simulink subsystem "ctrl_ez_sub"  (R2024b)
settings: Solver=VariableStepAuto  StartTime=0.0  StopTime=10.0  RelTol=1e-3
values from neighbouring files (symbols this model uses):
  t_ss = tsw/30    (= 5.12820512821e-07)    [fidelity_pfc_vals.m]
  tsw = 1/(fsw*1e3)    (= 1.53846153846e-05)    [fidelity_pfc_vals.m]
undefined symbols (not defined in the file or in its folder): Discrete, Fc, spsSVPWMGenerator2LevelModel
libraries: mcbcontrolslib x5, slpidlib x4, simulink x4, simulink_extras x1, dspswit3 x1
settings Model: Creator=Angel  LastModifiedBy=Angel

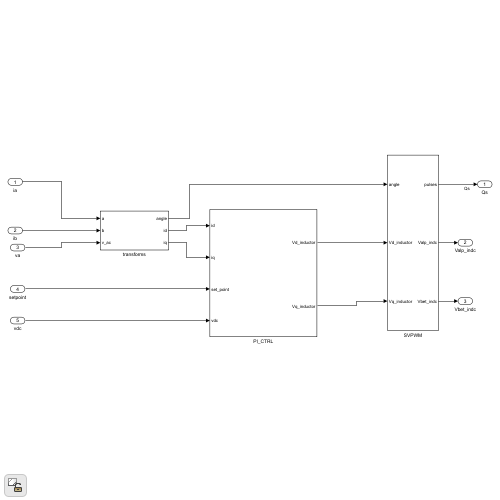
[thumbnail: Simulink's stored preview of the top-level diagram]
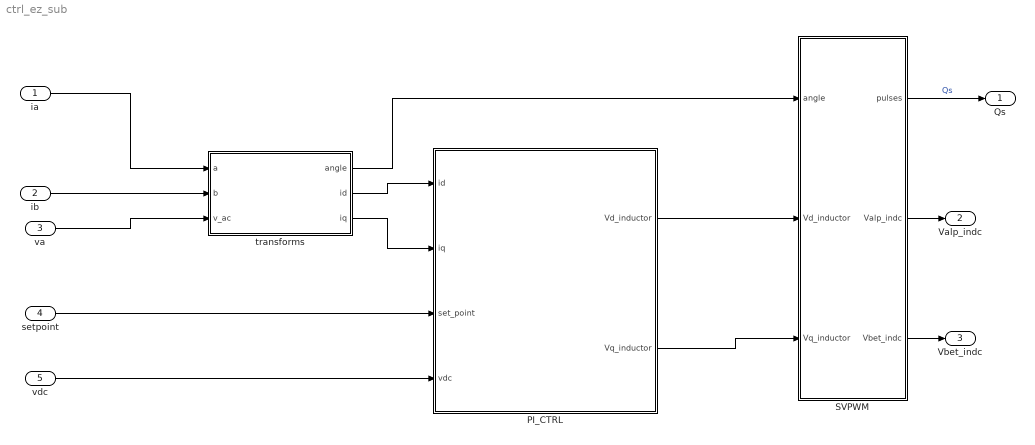
== system ctrl_ez_sub ==
  ia : Inport  OutDataTypeStr=single
  ib : Inport  Port=2  OutDataTypeStr=single
  va : Inport  Port=3  OutDataTypeStr=single
  setpoint : Inport  Port=4  OutDataTypeStr=single
  vdc : Inport  Port=5  OutDataTypeStr=single
  PI_CTRL : Subsystem  SystemSampleTime=tsw
  SVPWM : Subsystem  SystemSampleTime=tsw
  transforms : Subsystem  SystemSampleTime=tsw
  Qs : Outport
  Valp_indc : Outport  Port=2
  Vbet_indc : Outport  Port=3
  wires:
  SVPWM/1(pulses) -> Qs/1  "Qs"
  PI_CTRL/2(Vq_inductor) -> SVPWM/3(Vq_inductor)
  PI_CTRL/1(Vd_inductor) -> SVPWM/2(Vd_inductor)
  setpoint/1 -> PI_CTRL/3(set_point)
  transforms/2(id) -> PI_CTRL/1(id)
  transforms/1(angle) -> SVPWM/1(angle)
  transforms/3(iq) -> PI_CTRL/2(iq)
  va/1 -> transforms/3(v_ac)
  ib/1 -> transforms/2(b)
  ia/1 -> transforms/1(a)
  vdc/1 -> PI_CTRL/4(vdc)
  SVPWM/3(Vbet_indc) -> Vbet_indc/1
  SVPWM/2(Valp_indc) -> Valp_indc/1

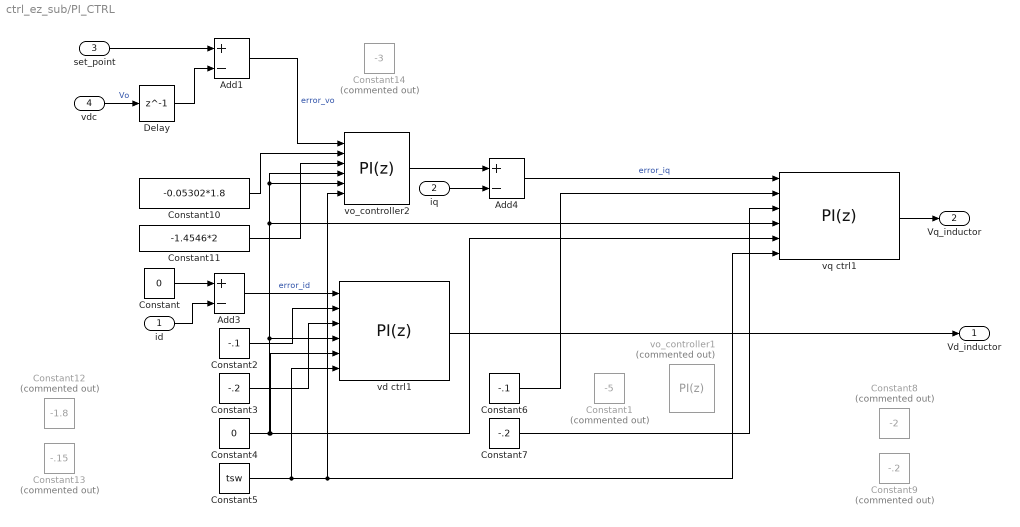
== system ctrl_ez_sub/PI_CTRL ==
  id : Inport
  iq : Inport  Port=2  OutDataTypeStr=single
  set_point : Inport  Port=3
  vdc : Inport  Port=4
  Add1 : Sum  Inputs=+-
  Add3 : Sum  Inputs=+-
  Add4 : Sum  Inputs=+-
  Constant : Constant  Value=0  OutDataTypeStr=single  SampleTime=-1
  Constant1 : Constant  Commented=on  Value=-5  SampleTime=t_ss
  Constant10 : Constant  Value=-0.05302*1.8  OutDataTypeStr=single  SampleTime=-1
  Constant11 : Constant  Value=-1.4546*2  OutDataTypeStr=single  SampleTime=-1
  Constant12 : Constant  Commented=on  Value=-1.8  OutDataTypeStr=single  SampleTime=-1
  Constant13 : Constant  Commented=on  Value=-.15  OutDataTypeStr=single  SampleTime=-1
  Constant14 : Constant  Commented=on  Value=-3  OutDataTypeStr=single  SampleTime=-1
  Constant2 : Constant  Value=-.1  OutDataTypeStr=single  SampleTime=-1
  Constant3 : Constant  Value=-.2  OutDataTypeStr=single  SampleTime=-1
  Constant4 : Constant  Value=0  OutDataTypeStr=single  SampleTime=-1
  Constant5 : Constant  Value=tsw  OutDataTypeStr=single  SampleTime=-1
  Constant6 : Constant  Value=-.1  OutDataTypeStr=single  SampleTime=-1
  Constant7 : Constant  Value=-.2  OutDataTypeStr=single  SampleTime=-1
  Constant8 : Constant  Commented=on  Value=-2  OutDataTypeStr=single  SampleTime=-1
  Constant9 : Constant  Commented=on  Value=-.2  OutDataTypeStr=single  SampleTime=-1
  Delay : Delay  DelayLength=1  InitialCondition=580
  "vd ctrl1 " : slpidlib/PID Controller  Controller=PI  Form=Parallel  TimeDomain=Discrete-time  UseExternalTs=on  SampleTime=-1  IntegratorMethod=Forward Euler  FilterMethod=Forward Euler  ControllerParametersSource=external  P=1  I=1  UseKiTs=off  D=0  UseExternalDerivativeSource=off  N=100  UseFilter=on  TunerSelectOption=Transfer Function Based (PID Tuner App)  ZeroCross=off  InitialConditionSource=external  InitialConditionForIntegrator=0  InitialConditionForFilter=0  DifferentiatorICPrevScaledInput=0  ExternalReset=level  TrackingMode=off  Kt=1  LimitOutput=on  SatLimitsSource=internal  UpperSaturationLimit=50  LowerSaturationLimit=-50  LinearizeAsGain=on  AntiWindupMode=clamping  Kb=1  LimitIntegrator=off  UpperIntegratorSaturationLimit=inf  LowerIntegratorSaturationLimit=-inf  RndMeth=Simplest  POutMin=[]  POutMax=[]  IOutMin=[]  IOutMax=[]  DOutMin=[]  DOutMax=[]  NOutMin=[]  NOutMax=[]  SumOutMin=[]  SumOutMax=[]  SaturationOutDataTypeStr=Inherit: Inherit via back propagation  SaturationOutMin=[]  SaturationOutMax=[]  PParamMin=[]  PParamMax=[]  IParamMin=[]  IParamMax=[]  DParamMin=[]  DParamMax=[]  NParamMin=[]  NParamMax=[]  KbParamMin=[]  KbParamMax=[]  KtParamMin=[]  KtParamMax=[]  KbOutMin=[]  KbOutMax=[]  KtOutMin=[]  KtOutMax=[]  IntegratorOutMin=[]  IntegratorOutMax=[]  FilterOutMin=[]  FilterOutMax=[]  SumI1OutMin=[]  SumI1OutMax=[]  SumI2OutMin=[]  SumI2OutMax=[]  SumI3OutMin=[]  SumI3OutMax=[]  SumI4OutMin=[]  SumI4OutMax=[]  SumDOutMin=[]  SumDOutMax=[]  DifferentiatorOutMin=[]  DifferentiatorOutMax=[]  FilterDiffOutCoefMin=[]  FilterDiffOutCoefMax=[]  ReciprocalOutMin=[]  ReciprocalOutMax=[]  SumDenOutMin=[]  SumDenOutMax=[]  SumNumOutMin=[]  SumNumOutMax=[]  DivideOutMin=[]  DivideOutMax=[]  UdiffTsProdOutMin=[]  UdiffTsProdOutMax=[]  NTsProdOutMin=[]  NTsProdOutMax=[]  UintegralTsProdOutMin=[]  UintegralTsProdOutMax=[]  UngainTsProdOutMin=[]  UngainTsProdOutMax=[]  ClampingZeroOutDataTypeStr=Inherit: Inherit via back propagation  ClampingZeroOutMin=[]  ClampingZeroOutMax=[]  FilterDenConstantOutDataTypeStr=Inherit: Inherit via back propagation  FilterDenConstantOutMin=[]  FilterDenConstantOutMax=[]  PCopyOutDataTypeStr=Inherit: Inherit via back propagation  PCopyOutMin=[]  PCopyOutMax=[]  NCopyOutDataTypeStr=Inherit: Inherit via back propagation  NCopyOutMin=[]  NCopyOutMax=[]  IntegratorContinuousStateAttributes=''  IntegratorStateMustResolveToSignalObject=off  IntegratorRTWStateStorageClass=Auto  FilterContinuousStateAttributes=''  FilterStateMustResolveToSignalObject=off  FilterRTWStateStorageClass=Auto  ParallelPVariant=ExternalParameters  IdealPVariant=Disabled  IVariant=ExternalParameters  DVariant=Disabled  IntegratorVariant=Discrete  SatVariant=Enabled  AWVariant=DiscClampingParallel  PCopyVariant=Disabled  TRVariant=Disabled  FdbkBlocksVariant=Forward  IdealPFdbkVariant=Disabled  SatFdbkVariant=Disabled  DerivativeFilterVariant=Disabled  NVariant=Disabled  NCopyVariant=Disabled_SignalSpec  FilterICVariant=Disabled  IntegratorICVariant=ExternalICs  ExternalResetVariant=ExternalReset  TRSumVariant=Passthrough  SumFdbkVariant=Disabled  SumVariant=Sum_PI  TsampFilterVariant=InternalTs  TsampNgainVariant=Passthrough  TsampIntegralVariant=ExternalTs  ExternalSaturationOutDataTypeStr=Inherit: Same as second input  DerivativeSourceVariant=Disabled  PreIntVariant=InternalPreInt
  vo_controller1 : slpidlib/PID Controller  Commented=on  Controller=PI  Form=Parallel  TimeDomain=Discrete-time  UseExternalTs=off  SampleTime=-1  IntegratorMethod=Forward Euler  FilterMethod=Forward Euler  ControllerParametersSource=internal  P=-0.053025  I=-1.4546  UseKiTs=off  D=0  UseExternalDerivativeSource=off  N=100  UseFilter=on  TunerSelectOption=Transfer Function Based (PID Tuner App)  InitialConditionSource=internal  InitialConditionForIntegrator=0  InitialConditionForFilter=0  DifferentiatorICPrevScaledInput=0  ExternalReset=none  TrackingMode=off  Kt=1  LimitOutput=off  SatLimitsSource=internal  UpperSaturationLimit=inf  LowerSaturationLimit=0  LinearizeAsGain=on  AntiWindupMode=clamping  Kb=1  LimitIntegrator=off  UpperIntegratorSaturationLimit=inf  LowerIntegratorSaturationLimit=-inf  POutMin=[]  POutMax=[]  IOutMin=[]  IOutMax=[]  DOutMin=[]  DOutMax=[]  NOutMin=[]  NOutMax=[]  SumOutMin=[]  SumOutMax=[]  SaturationOutMin=[]  SaturationOutMax=[]  PParamMin=[]  PParamMax=[]  IParamMin=[]  IParamMax=[]  DParamMin=[]  DParamMax=[]  NParamMin=[]  NParamMax=[]  KbParamMin=[]  KbParamMax=[]  KtParamMin=[]  KtParamMax=[]  KbOutMin=[]  KbOutMax=[]  KtOutMin=[]  KtOutMax=[]  IntegratorOutMin=[]  IntegratorOutMax=[]  FilterOutMin=[]  FilterOutMax=[]  SumI1OutMin=[]  SumI1OutMax=[]  SumI2OutMin=[]  SumI2OutMax=[]  SumI3OutMin=[]  SumI3OutMax=[]  SumI4OutMin=[]  SumI4OutMax=[]  SumDOutMin=[]  SumDOutMax=[]  DifferentiatorOutMin=[]  DifferentiatorOutMax=[]  FilterDiffOutCoefMin=[]  FilterDiffOutCoefMax=[]  ReciprocalOutMin=[]  ReciprocalOutMax=[]  SumDenOutMin=[]  SumDenOutMax=[]  SumNumOutMin=[]  SumNumOutMax=[]  DivideOutMin=[]  DivideOutMax=[]  UdiffTsProdOutMin=[]  UdiffTsProdOutMax=[]  NTsProdOutMin=[]  NTsProdOutMax=[]  UintegralTsProdOutMin=[]  UintegralTsProdOutMax=[]  UngainTsProdOutMin=[]  UngainTsProdOutMax=[]  ClampingZeroOutDataTypeStr=Inherit: Inherit via back propagation  ClampingZeroOutMin=[]  ClampingZeroOutMax=[]  FilterDenConstantOutDataTypeStr=Inherit: Inherit via back propagation  FilterDenConstantOutMin=[]  FilterDenConstantOutMax=[]  PCopyOutDataTypeStr=Inherit: Inherit via back propagation  PCopyOutMin=[]  PCopyOutMax=[]  NCopyOutDataTypeStr=Inherit: Inherit via back propagation  NCopyOutMin=[]  NCopyOutMax=[]  IntegratorContinuousStateAttributes=''  IntegratorStateMustResolveToSignalObject=off  IntegratorRTWStateStorageClass=Auto  FilterContinuousStateAttributes=''  FilterStateMustResolveToSignalObject=off  FilterRTWStateStorageClass=Auto  ParallelPVariant=InternalParameters  IdealPVariant=Disabled  IVariant=InternalParameters  DVariant=Disabled  IntegratorVariant=Discrete  SatVariant=Disabled  AWVariant=Passthrough  PCopyVariant=Disabled  TRVariant=Disabled  FdbkBlocksVariant=Forward  IdealPFdbkVariant=Disabled  SatFdbkVariant=Disabled  DerivativeFilterVariant=Disabled  NVariant=Disabled  NCopyVariant=Disabled_SignalSpec  FilterICVariant=Disabled  IntegratorICVariant=InternalICs  ExternalResetVariant=Disabled  TRSumVariant=Passthrough  SumFdbkVariant=Disabled  SumVariant=Sum_PI  TsampFilterVariant=InternalTs  TsampNgainVariant=Passthrough  TsampIntegralVariant=Disabled_SignalSpec  ExternalSaturationOutDataTypeStr=Inherit: Same as second input  DerivativeSourceVariant=Disabled  PreIntVariant=InternalPreInt
  vo_controller2 : slpidlib/PID Controller  Controller=PI  Form=Parallel  TimeDomain=Discrete-time  UseExternalTs=on  SampleTime=-1  IntegratorMethod=Forward Euler  FilterMethod=Forward Euler  ControllerParametersSource=external  P=-0.053025  I=-1.4546  UseKiTs=off  D=0  UseExternalDerivativeSource=off  N=100  UseFilter=on  TunerSelectOption=Transfer Function Based (PID Tuner App)  InitialConditionSource=external  InitialConditionForIntegrator=0  InitialConditionForFilter=0  DifferentiatorICPrevScaledInput=0  ExternalReset=level  TrackingMode=off  Kt=1  LimitOutput=on  SatLimitsSource=internal  UpperSaturationLimit=300  LowerSaturationLimit=-300  LinearizeAsGain=on  AntiWindupMode=clamping  Kb=1  LimitIntegrator=off  UpperIntegratorSaturationLimit=inf  LowerIntegratorSaturationLimit=-inf  POutMin=[]  POutMax=[]  IOutMin=[]  IOutMax=[]  DOutMin=[]  DOutMax=[]  NOutMin=[]  NOutMax=[]  SumOutMin=[]  SumOutMax=[]  SaturationOutMin=[]  SaturationOutMax=[]  PParamMin=[]  PParamMax=[]  IParamMin=[]  IParamMax=[]  DParamMin=[]  DParamMax=[]  NParamMin=[]  NParamMax=[]  KbParamMin=[]  KbParamMax=[]  KtParamMin=[]  KtParamMax=[]  KbOutMin=[]  KbOutMax=[]  KtOutMin=[]  KtOutMax=[]  IntegratorOutMin=[]  IntegratorOutMax=[]  FilterOutMin=[]  FilterOutMax=[]  SumI1OutMin=[]  SumI1OutMax=[]  SumI2OutMin=[]  SumI2OutMax=[]  SumI3OutMin=[]  SumI3OutMax=[]  SumI4OutMin=[]  SumI4OutMax=[]  SumDOutMin=[]  SumDOutMax=[]  DifferentiatorOutMin=[]  DifferentiatorOutMax=[]  FilterDiffOutCoefMin=[]  FilterDiffOutCoefMax=[]  ReciprocalOutMin=[]  ReciprocalOutMax=[]  SumDenOutMin=[]  SumDenOutMax=[]  SumNumOutMin=[]  SumNumOutMax=[]  DivideOutMin=[]  DivideOutMax=[]  UdiffTsProdOutMin=[]  UdiffTsProdOutMax=[]  NTsProdOutMin=[]  NTsProdOutMax=[]  UintegralTsProdOutMin=[]  UintegralTsProdOutMax=[]  UngainTsProdOutMin=[]  UngainTsProdOutMax=[]  ClampingZeroOutDataTypeStr=Inherit: Inherit via back propagation  ClampingZeroOutMin=[]  ClampingZeroOutMax=[]  FilterDenConstantOutDataTypeStr=Inherit: Inherit via back propagation  FilterDenConstantOutMin=[]  FilterDenConstantOutMax=[]  PCopyOutDataTypeStr=Inherit: Inherit via back propagation  PCopyOutMin=[]  PCopyOutMax=[]  NCopyOutDataTypeStr=Inherit: Inherit via back propagation  NCopyOutMin=[]  NCopyOutMax=[]  IntegratorContinuousStateAttributes=''  IntegratorStateMustResolveToSignalObject=off  IntegratorRTWStateStorageClass=Auto  FilterContinuousStateAttributes=''  FilterStateMustResolveToSignalObject=off  FilterRTWStateStorageClass=Auto  ParallelPVariant=ExternalParameters  IdealPVariant=Disabled  IVariant=ExternalParameters  DVariant=Disabled  IntegratorVariant=Discrete  SatVariant=Enabled  AWVariant=DiscClampingParallel  PCopyVariant=Disabled  TRVariant=Disabled  FdbkBlocksVariant=Forward  IdealPFdbkVariant=Disabled  SatFdbkVariant=Disabled  DerivativeFilterVariant=Disabled  NVariant=Disabled  NCopyVariant=Disabled_SignalSpec  FilterICVariant=Disabled  IntegratorICVariant=ExternalICs  ExternalResetVariant=ExternalReset  TRSumVariant=Passthrough  SumFdbkVariant=Disabled  SumVariant=Sum_PI  TsampFilterVariant=InternalTs  TsampNgainVariant=Passthrough  TsampIntegralVariant=ExternalTs  ExternalSaturationOutDataTypeStr=Inherit: Same as second input  DerivativeSourceVariant=Disabled  PreIntVariant=InternalPreInt
  "vq ctrl1 " : slpidlib/PID Controller  Controller=PI  Form=Parallel  TimeDomain=Discrete-time  UseExternalTs=on  SampleTime=-1  IntegratorMethod=Forward Euler  FilterMethod=Forward Euler  ControllerParametersSource=external  P=1  I=1  UseKiTs=off  D=0  UseExternalDerivativeSource=off  N=100  UseFilter=on  TunerSelectOption=Transfer Function Based (PID Tuner App)  ZeroCross=off  InitialConditionSource=external  InitialConditionForIntegrator=0  InitialConditionForFilter=0  DifferentiatorICPrevScaledInput=0  ExternalReset=level  TrackingMode=off  Kt=1  LimitOutput=on  SatLimitsSource=internal  UpperSaturationLimit=50  LowerSaturationLimit=-50  LinearizeAsGain=on  AntiWindupMode=clamping  Kb=1  LimitIntegrator=off  UpperIntegratorSaturationLimit=inf  LowerIntegratorSaturationLimit=-inf  RndMeth=Simplest  POutMin=[]  POutMax=[]  IOutMin=[]  IOutMax=[]  DOutMin=[]  DOutMax=[]  NOutMin=[]  NOutMax=[]  SumOutMin=[]  SumOutMax=[]  SaturationOutDataTypeStr=Inherit: Inherit via back propagation  SaturationOutMin=[]  SaturationOutMax=[]  PParamMin=[]  PParamMax=[]  IParamMin=[]  IParamMax=[]  DParamMin=[]  DParamMax=[]  NParamMin=[]  NParamMax=[]  KbParamMin=[]  KbParamMax=[]  KtParamMin=[]  KtParamMax=[]  KbOutMin=[]  KbOutMax=[]  KtOutMin=[]  KtOutMax=[]  IntegratorOutMin=[]  IntegratorOutMax=[]  FilterOutMin=[]  FilterOutMax=[]  SumI1OutMin=[]  SumI1OutMax=[]  SumI2OutMin=[]  SumI2OutMax=[]  SumI3OutMin=[]  SumI3OutMax=[]  SumI4OutMin=[]  SumI4OutMax=[]  SumDOutMin=[]  SumDOutMax=[]  DifferentiatorOutMin=[]  DifferentiatorOutMax=[]  FilterDiffOutCoefMin=[]  FilterDiffOutCoefMax=[]  ReciprocalOutMin=[]  ReciprocalOutMax=[]  SumDenOutMin=[]  SumDenOutMax=[]  SumNumOutMin=[]  SumNumOutMax=[]  DivideOutMin=[]  DivideOutMax=[]  UdiffTsProdOutMin=[]  UdiffTsProdOutMax=[]  NTsProdOutMin=[]  NTsProdOutMax=[]  UintegralTsProdOutMin=[]  UintegralTsProdOutMax=[]  UngainTsProdOutMin=[]  UngainTsProdOutMax=[]  ClampingZeroOutDataTypeStr=Inherit: Inherit via back propagation  ClampingZeroOutMin=[]  ClampingZeroOutMax=[]  FilterDenConstantOutDataTypeStr=Inherit: Inherit via back propagation  FilterDenConstantOutMin=[]  FilterDenConstantOutMax=[]  PCopyOutDataTypeStr=Inherit: Inherit via back propagation  PCopyOutMin=[]  PCopyOutMax=[]  NCopyOutDataTypeStr=Inherit: Inherit via back propagation  NCopyOutMin=[]  NCopyOutMax=[]  IntegratorContinuousStateAttributes=''  IntegratorStateMustResolveToSignalObject=off  IntegratorRTWStateStorageClass=Auto  FilterContinuousStateAttributes=''  FilterStateMustResolveToSignalObject=off  FilterRTWStateStorageClass=Auto  ParallelPVariant=ExternalParameters  IdealPVariant=Disabled  IVariant=ExternalParameters  DVariant=Disabled  IntegratorVariant=Discrete  SatVariant=Enabled  AWVariant=DiscClampingParallel  PCopyVariant=Disabled  TRVariant=Disabled  FdbkBlocksVariant=Forward  IdealPFdbkVariant=Disabled  SatFdbkVariant=Disabled  DerivativeFilterVariant=Disabled  NVariant=Disabled  NCopyVariant=Disabled_SignalSpec  FilterICVariant=Disabled  IntegratorICVariant=ExternalICs  ExternalResetVariant=ExternalReset  TRSumVariant=Passthrough  SumFdbkVariant=Disabled  SumVariant=Sum_PI  TsampFilterVariant=InternalTs  TsampNgainVariant=Passthrough  TsampIntegralVariant=ExternalTs  ExternalSaturationOutDataTypeStr=Inherit: Same as second input  DerivativeSourceVariant=Disabled  PreIntVariant=InternalPreInt
  Vd_inductor : Outport
  Vq_inductor : Outport  Port=2
  wires:
  vo_controller2/1 -> Add4/1
  "vq ctrl1 "/1 -> Vq_inductor/1
  "vd ctrl1 "/1 -> Vd_inductor/1
  Constant3/1 -> "vd ctrl1 "/3
  Constant5/1 -> "vd ctrl1 "/6, vo_controller2/6, "vq ctrl1 "/6
  Constant7/1 -> "vq ctrl1 "/3
  Constant2/1 -> "vd ctrl1 "/2
  Constant4/1 -> "vd ctrl1 "/4, "vq ctrl1 "/4, vo_controller2/4, vo_controller2/5, "vq ctrl1 "/5, "vd ctrl1 "/5
  Constant6/1 -> "vq ctrl1 "/2
  id/1 -> Add3/2
  Constant10/1 -> vo_controller2/2
  Constant/1 -> Add3/1
  Constant11/1 -> vo_controller2/3
  Add3/1 -> "vd ctrl1 "/1  "error_id"
  Add4/1 -> "vq ctrl1 "/1  "error_iq"
  Delay/1 -> Add1/2
  set_point/1 -> Add1/1
  Add1/1 -> vo_controller2/1  "error_vo"
  vdc/1 -> Delay/1  "Vo"
  iq/1 -> Add4/2

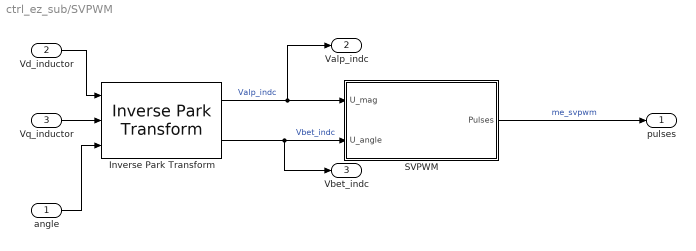
== system ctrl_ez_sub/SVPWM ==
  angle : Inport
  Vd_inductor : Inport  Port=2
  Vq_inductor : Inport  Port=3
  Inverse Park Transform : mcbcontrolslib/Inverse Park Transform  PhaseInput=Two inputs  AxisAlignment=D-axis  ThetaInput=Electrical position  AngleInput=Radians  N_points=1024
  SVPWM : Subsystem  AncestorBlock=spsSVPWMGenerator2LevelModel/Discrete
  pulses : Outport
  Valp_indc : Outport  Port=2
  Vbet_indc : Outport  Port=3
  wires:
  SVPWM/1(Pulses) -> pulses/1  "me_svpwm"
  Inverse Park Transform/2 -> SVPWM/2(U_angle), Vbet_indc/1  "Vbet_indc"
  Inverse Park Transform/1 -> SVPWM/1(U_mag), Valp_indc/1  "Valp_indc"
  angle/1 -> Inverse Park Transform/3
  Vq_inductor/1 -> Inverse Park Transform/2
  Vd_inductor/1 -> Inverse Park Transform/1

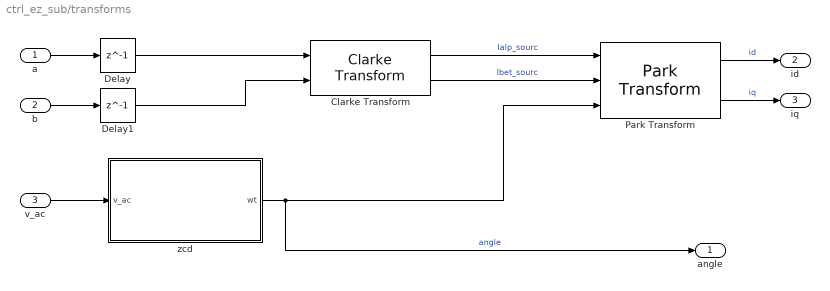
== system ctrl_ez_sub/transforms ==
  a : Inport
  b : Inport  Port=2
  v_ac : Inport  Port=3
  Clarke Transform : mcbcontrolslib/Clarke Transform  VariantControl=Variant2  PhaseInput=Two inputs  EnPowerInv=off
  Delay : Delay  DelayLength=1
  Delay1 : Delay  DelayLength=1
  Park Transform : mcbcontrolslib/Park Transform  PhaseInput=Two inputs  AxisAlignment=D-axis  ThetaInput=Electrical position  AngleInput=Radians  N_points=4095
  zcd : Subsystem  SystemSampleTime=tsw
  angle : Outport
  id : Outport  Port=2
  iq : Outport  Port=3
  wires:
  Delay1/1 -> Clarke Transform/2
  Delay/1 -> Clarke Transform/1
  Park Transform/2 -> iq/1  "iq"
  Park Transform/1 -> id/1  "id"
  zcd/1(wt) -> Park Transform/3, angle/1  "angle"
  b/1 -> Delay1/1
  a/1 -> Delay/1
  v_ac/1 -> zcd/1(v_ac)
  Clarke Transform/2 -> Park Transform/2  "Ibet_sourc"
  Clarke Transform/1 -> Park Transform/1  "Ialp_sourc"

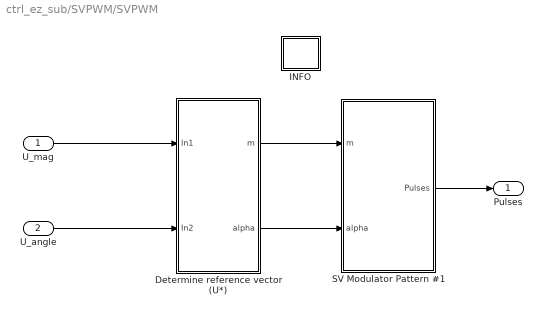
== system ctrl_ez_sub/SVPWM/SVPWM ==
  U_mag : Inport  OutDataTypeStr=single
  U_angle : Inport  Port=2  OutDataTypeStr=single
  Determine reference vector (U*) : Subsystem
  INFO : Subsystem
      mask Display: disp('?')
  SV Modulator Pattern #1 : Subsystem
  Pulses : Outport
  wires:
  Determine reference vector (U*)/2(alpha) -> SV Modulator Pattern #1/2(alpha)
  Determine reference vector (U*)/1(m) -> SV Modulator Pattern #1/1(m)
  SV Modulator Pattern #1/1(Pulses) -> Pulses/1
  U_angle/1 -> Determine reference vector (U*)/2(In2)
  U_mag/1 -> Determine reference vector (U*)/1(In1)

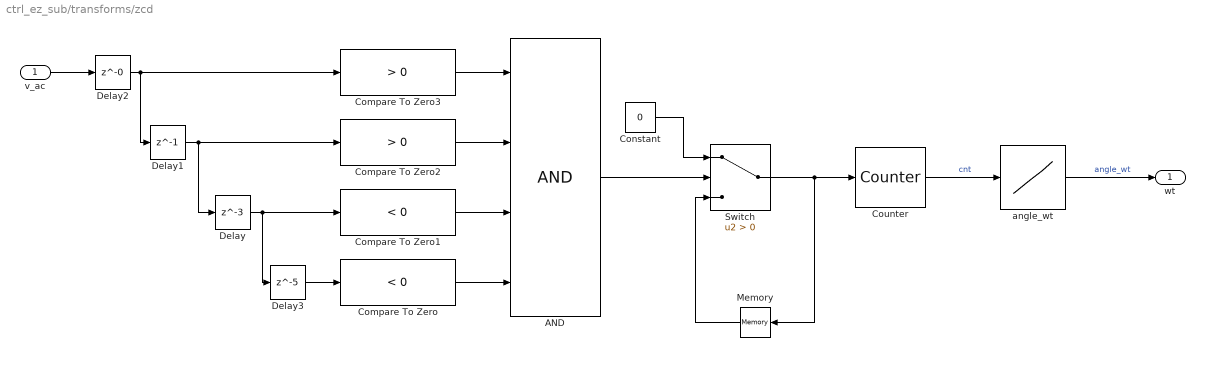
== system ctrl_ez_sub/transforms/zcd ==
  v_ac : Inport  OutDataTypeStr=single
  AND : Logic  Inputs=4  AllPortsSameDT=off  OutDataTypeStr=boolean
  Compare To Zero : simulink/Logic and Bit Operations/Compare To Zero  relop=<  OutDataTypeStr=boolean
  Compare To Zero1 : simulink/Logic and Bit Operations/Compare To Zero  relop=<  OutDataTypeStr=boolean
  Compare To Zero2 : simulink/Logic and Bit Operations/Compare To Zero  relop=>  OutDataTypeStr=boolean
  Compare To Zero3 : simulink/Logic and Bit Operations/Compare To Zero  relop=>  OutDataTypeStr=boolean
  Constant : Constant  Value=0  OutDataTypeStr=boolean  SampleTime=-1
  Counter : dspswit3/Counter  Direction=Up  CountEvent=Free running  CounterSize=User defined  MaxCount=(.02/tsw)+1  InitialCount=0  Output=Count  HitValue=32  ResetInput=on  SamplesPerFrame=1  Ts=-1  CntDtype=uint32  HitDtype=Logical
  Delay : Delay  DelayLength=3
  Delay1 : Delay  DelayLength=1
  Delay2 : Delay  DelayLength=0
  Delay3 : Delay  DelayLength=5
  Memory : Memory  InitialCondition=1  InheritSampleTime=on
  Switch : Switch  Criteria=u2 > Threshold  SaturateOnIntegerOverflow=off  InputSameDT=off
  angle_wt : Lookup_n-D  NumberOfTableDimensions=1  BreakpointsForDimension1=0:.02/tsw  IndexSearchMethod=Evenly spaced points  Table=0:pi*2/(.02/tsw):2*pi;  TableDataTypeStr=single  InterpMethod=Flat  InternalRulePriority=Speed  OutDataTypeStr=single
  wt : Outport
  wires:
  Counter/1 -> angle_wt/1  "cnt"
  Constant/1 -> Switch/1
  Memory/1 -> Switch/3
  AND/1 -> Switch/2
  Switch/1 -> Counter/1, Memory/1
  Compare To Zero2/1 -> AND/2
  Compare To Zero/1 -> AND/4
  Compare To Zero1/1 -> AND/3
  Compare To Zero3/1 -> AND/1
  Delay1/1 -> Delay/1, Compare To Zero2/1
  Delay2/1 -> Delay1/1, Compare To Zero3/1
  Delay/1 -> Compare To Zero1/1, Delay3/1
  Delay3/1 -> Compare To Zero/1
  v_ac/1 -> Delay2/1
  angle_wt/1 -> wt/1  "angle_wt"

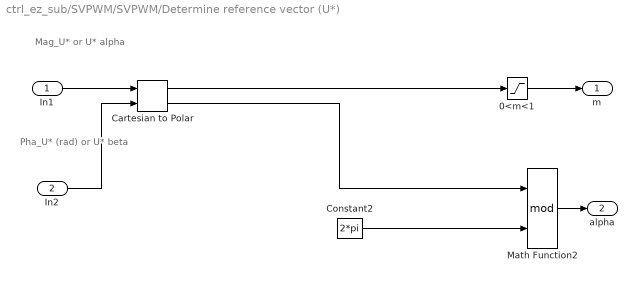
== system ctrl_ez_sub/SVPWM/SVPWM/Determine reference vector (U*) ==
  note: Pha_U* (rad)
      | or
      | U* beta
  note: Mag_U*
      | or
      | U* alpha
  In1 : Inport
  In2 : Inport  Port=2
  "0<m<1 " : Saturate  UpperLimit=1  LowerLimit=0  OutDataTypeStr=single
  Cartesian to Polar : simulink_extras/Transformations/Cartesian to Polar
  Constant2 : Constant  Value=2*pi  OutDataTypeStr=single  SampleTime=-1
  Math Function2 : Math  Operator=mod  SignedPower=on
  m : Outport
  alpha : Outport  Port=2
  wires:
  Math Function2/1 -> alpha/1
  Constant2/1 -> Math Function2/2
  Cartesian to Polar/2 -> Math Function2/1
  Cartesian to Polar/1 -> "0<m<1 "/1
  In2/1 -> Cartesian to Polar/2
  In1/1 -> Cartesian to Polar/1
  "0<m<1 "/1 -> m/1

== system ctrl_ez_sub/SVPWM/SVPWM/INFO ==
  note: Pattern #2:
      | With this pattern, identified as "Hardware-Determined" by Texas Instruments, there is always one PWM channel staying constant for the entire PWM period.
      |  So the number of switching times for this pattern is less than pattern #1. As a result, switching losses will be reduced with Pattern #2.
  note: Pattern #1:
      | With this pattern, identified as "Software-Determined" by Texas Instruments, each PWM channel switches twice per every PWM period.
  note: --------------------------------------------------------------------------------------------------------------------------------------------------------------------
  note: Reference: Application Report SPRA524
      | Space-Vector PWM with TMS320C24x Using H/W & S/W Determined Switching Patterns
      | Zhenyu Yu, Texas Instruments
  note: The objective of the SV PWM technique is to approximate the reference voltage vector (U*) instantaneously
      | by combination of the switching states corresponding to the basic space vectors.
  note: U7 = 1 1 1
  note: Q1 Q3 Q5
  note: --------------------------------------------------------
  note: Three-Phase VSC Diagram
  note: -
  note: +
  note: --------------------------------------------------------
  note: |
      | |
      | |
  note: ---Vc
  note: |
      | |
      | |
  note: |
      | |
      | |
      | |
      | |
      | |
  note: [Q6]
  note: [Q5]
  note: |
      | |
      | |
  note: ---Vb
  note: |
      | |
      | |
  note: |
      | |
      | |
      | |
      | |
      | |
  note: [Q4]
  note: [Q3]
  note: |
      | |
      | |
  note: ---Va
  note: |
      | |
      | |
  note: |
      | |
      | |
      | |
      | |
      | |
  note: [Q2]
  note: [Q1]
  note: Vdc
  note: [n] = Sector number
  note: [2]
  note: Basic Space Vectors and Switching States
  note: U4 = 0 1 1
  note: U5 = 0 0 1
  note: U6 = 1 0 1
  note: U0 = 0 0 0
  note: U3 = 0 1 0
  note: U2 = 1 1 0
  note: U1 = 1 0 0
  note: [6]
  note: [5]
  note: [4]
  note: [3]
  note: [1]
  note: 3                       2
      |       3                   2
      |         3               2
      |           3           2
      |             3       2
      |               3   2
      | 4 4 4 4 4 4 4 4 0 1 1 1 1 1 1 1 1
      |               5   6
      |             5       6
      |           5           6
      |         5               6
      |       5                   6
      |     5                       6
  note: Two symmetrical switching patterns have been implemented:

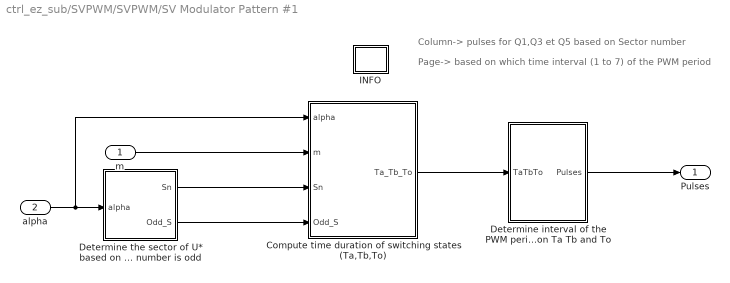
== system ctrl_ez_sub/SVPWM/SVPWM/SV Modulator Pattern #1 ==
  note: Page-> based on which time interval (1 to 7) of the PWM period
  note: Column-> pulses for Q1,Q3 et Q5 based on Sector number
  m : Inport
  alpha : Inport  Port=2
  "Compute time duration of switching states (Ta,Tb,To) " : Subsystem
  Determine interval of the PWM period based on Ta Tb and To : Subsystem
  "Determine the sector of U* based on alpha (rad). Also, determine if the sector number is odd" : Subsystem
  INFO : Subsystem
      mask Display: disp('?')
  Pulses : Outport
  wires:
  "Compute time duration of switching states (Ta,Tb,To) "/1(Ta_Tb_To) -> Determine interval of the PWM period based on Ta Tb and To/1(TaTbTo)
  m/1 -> "Compute time duration of switching states (Ta,Tb,To) "/2(m)
  alpha/1 -> "Compute time duration of switching states (Ta,Tb,To) "/1(alpha), "Determine the sector of U* based on alpha (rad). Also, determine if the sector number is odd"/1(alpha)
  Determine interval of the PWM period based on Ta Tb and To/1(Pulses) -> Pulses/1
  "Determine the sector of U* based on alpha (rad). Also, determine if the sector number is odd"/2(Odd_S) -> "Compute time duration of switching states (Ta,Tb,To) "/4(Odd_S)
  "Determine the sector of U* based on alpha (rad). Also, determine if the sector number is odd"/1(Sn) -> "Compute time duration of switching states (Ta,Tb,To) "/3(Sn)

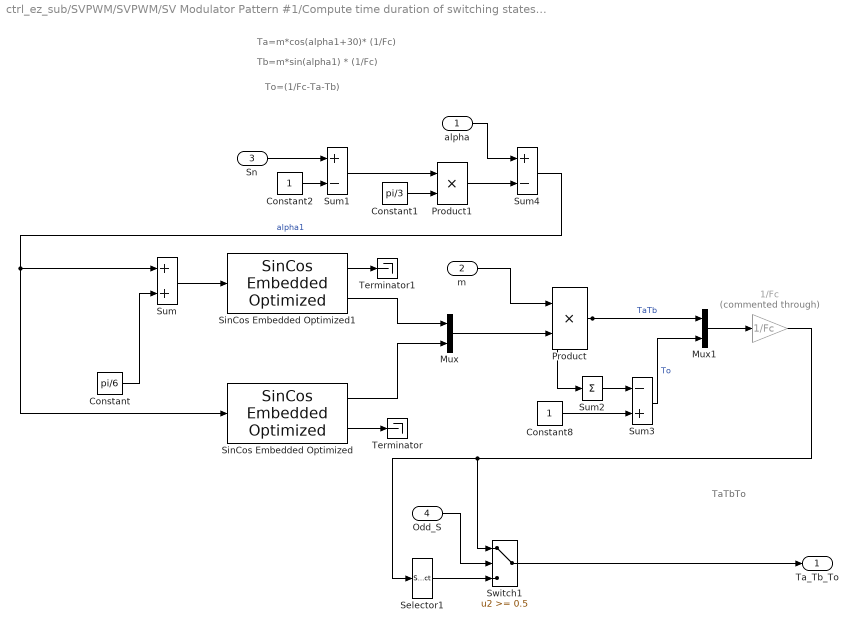
== system ctrl_ez_sub/SVPWM/SVPWM/SV Modulator Pattern #1/Compute time duration of switching states (Ta,Tb,To)  ==
  note: TaTbTo
  note: To=(1/Fc-Ta-Tb)
  note: Tb=m*sin(alpha1) * (1/Fc)
  note: Ta=m*cos(alpha1+30)* (1/Fc)
  alpha : Inport
  m : Inport  Port=2
  Sn : Inport  Port=3
  Odd_S : Inport  Port=4
  1/Fc : Gain  Commented=through  Gain=1/Fc  SaturateOnIntegerOverflow=on  OutDataTypeStr=Inherit: Same as input  ParamDataTypeStr=Inherit: Same as input
  Constant : Constant  Value=pi/6  OutDataTypeStr=single  SampleTime=-1
  Constant1 : Constant  Value=pi/3  OutDataTypeStr=single  SampleTime=-1
  Constant2 : Constant  OutDataTypeStr=single  SampleTime=-1
  Constant8 : Constant  OutDataTypeStr=single  SampleTime=-1
  Mux : Mux  Inputs=2
  Mux1 : Mux  Inputs=2
  Product : Product  OutDataTypeStr=single  SaturateOnIntegerOverflow=on
  Product1 : Product  SaturateOnIntegerOverflow=on  OutDataTypeStr=Inherit: Same as first input
  Selector1 : Selector  InputPortWidth=3  IndexOptions=Index vector (dialog)  Indices=[2 1 3]  OutputSizes=1
  SinCos Embedded Optimized : mcbcontrolslib/SinCos Embedded Optimized  LabelModeActiveChoice=MCB_Sin  OptforProc=off  ApproximationMethod=None  UserApproxMethod=Lookup  ApproxStatus=None  InterpMethod=Linear point-slope  NumberOfDataPoints=16  NumberOfIterations=11  RemoveProtectionAgainstOutOfRangeInput=off  TableDataTypeStr=Inherit: Inherit via input  AngleInput=Radians  ThetaDataType=single  N_points=1024  DatatypeInput=Inherit from input  Datatype=Inherit: Same as input
  SinCos Embedded Optimized1 : mcbcontrolslib/SinCos Embedded Optimized  LabelModeActiveChoice=MCB_Sin  OptforProc=off  ApproximationMethod=None  UserApproxMethod=Lookup  ApproxStatus=None  InterpMethod=Linear point-slope  NumberOfDataPoints=16  NumberOfIterations=11  RemoveProtectionAgainstOutOfRangeInput=off  TableDataTypeStr=Inherit: Inherit via input  AngleInput=Radians  ThetaDataType=single  N_points=1024  DatatypeInput=Inherit from input  Datatype=Inherit: Same as input
  Sum : Sum  SaturateOnIntegerOverflow=on
  Sum1 : Sum  Inputs=+-  SaturateOnIntegerOverflow=on
  Sum2 : Sum  Inputs=1  SaturateOnIntegerOverflow=on
  Sum3 : Sum  Inputs=-+  SaturateOnIntegerOverflow=on
  Sum4 : Sum  Inputs=+-  SaturateOnIntegerOverflow=on
  Switch1 : Switch  Threshold=0.5  InputSameDT=off
  Terminator : Terminator
  Terminator1 : Terminator
  Ta_Tb_To : Outport
  wires:
  SinCos Embedded Optimized/1 -> Mux/2
  SinCos Embedded Optimized1/2 -> Mux/1
  SinCos Embedded Optimized1/1 -> Terminator1/1
  SinCos Embedded Optimized/2 -> Terminator/1
  Odd_S/1 -> Switch1/2
  Switch1/1 -> Ta_Tb_To/1
  Selector1/1 -> Switch1/3
  1/Fc/1 -> Switch1/1, Selector1/1
  Constant/1 -> Sum/2
  Sum4/1 -> Sum/1, SinCos Embedded Optimized/1  "alpha1"
  Mux1/1 -> 1/Fc/1
  Sum3/1 -> Mux1/2  "To"
  Product/1 -> Mux1/1, Sum2/1  "TaTb"
  alpha/1 -> Sum4/1
  Product1/1 -> Sum4/2
  Constant2/1 -> Sum1/2
  Sn/1 -> Sum1/1
  Constant1/1 -> Product1/2
  Sum1/1 -> Product1/1
  Constant8/1 -> Sum3/2
  Sum2/1 -> Sum3/1
  Sum/1 -> SinCos Embedded Optimized1/1
  m/1 -> Product/1
  Mux/1 -> Product/2

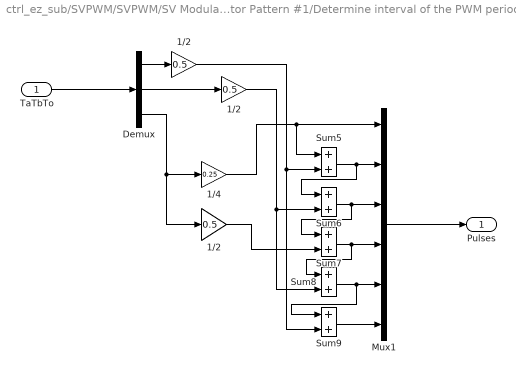
== system ctrl_ez_sub/SVPWM/SVPWM/SV Modulator Pattern #1/Determine interval of the PWM period based on Ta Tb and To ==
  TaTbTo : Inport
  "  1/2" : Gain  Gain=0.5  SaturateOnIntegerOverflow=on  OutDataTypeStr=Inherit: Same as input  ParamDataTypeStr=Inherit: Same as input
  " 1/2" : Gain  Gain=0.5  SaturateOnIntegerOverflow=on  OutDataTypeStr=Inherit: Same as input  ParamDataTypeStr=Inherit: Same as input
  " 1/2 " : Gain  Gain=0.5  SaturateOnIntegerOverflow=on  OutDataTypeStr=Inherit: Same as input  ParamDataTypeStr=Inherit: Same as input
  1/4 : Gain  Gain=0.25  SaturateOnIntegerOverflow=on  OutDataTypeStr=Inherit: Same as input  ParamDataTypeStr=Inherit: Same as input
  Demux : Demux  Outputs=3
      settings: DisplayOption=none
  Mux1 : Mux  Inputs=6
  Sum{5..9} (5 alike) : Sum  SaturateOnIntegerOverflow=on
  Pulses : Outport
  wires:
  Sum5/1 -> Sum6/1, Mux1/2
  Sum6/1 -> Sum7/1, Mux1/3
  Sum7/1 -> Sum8/1, Mux1/4
  Sum8/1 -> Sum9/1, Mux1/5
  Sum9/1 -> Mux1/6
  1/4/1 -> Sum5/1, Mux1/1
  Demux/1 -> " 1/2 "/1
  Demux/2 -> "  1/2"/1
  " 1/2"/1 -> Sum7/2
  TaTbTo/1 -> Demux/1
  "  1/2"/1 -> Sum8/2, Sum6/2
  Demux/3 -> " 1/2"/1, 1/4/1
  " 1/2 "/1 -> Sum9/2, Sum5/2
  Mux1/1 -> Pulses/1

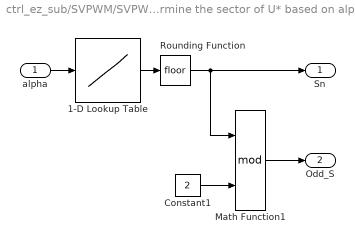
== system ctrl_ez_sub/SVPWM/SVPWM/SV Modulator Pattern #1/Determine the sector of U* based on alpha (rad). Also, determine if the sector number is odd ==
  alpha : Inport
  1-D Lookup Table : Lookup_n-D  NumberOfTableDimensions=1  BreakpointsForDimension1=single([0:pi/3:5*pi/3])  BeginIndexSearchUsingPreviousIndexResult=on  Table=single([1:6])  InternalRulePriority=Speed  RndMeth=Simplest
  Constant1 : Constant  Value=2  OutDataTypeStr=single  SampleTime=-1
  Math Function1 : Math  Operator=mod  SignedPower=on
  Rounding Function : Rounding
  Sn : Outport
  Odd_S : Outport  Port=2
  wires:
  alpha/1 -> 1-D Lookup Table/1
  Math Function1/1 -> Odd_S/1
  Constant1/1 -> Math Function1/2
  Rounding Function/1 -> Sn/1, Math Function1/1
  1-D Lookup Table/1 -> Rounding Function/1

== system ctrl_ez_sub/SVPWM/SVPWM/SV Modulator Pattern #1/INFO ==
  note: Interval 7
  note: Interval 6
  note: Interval 5
  note: Interval 4
  note: Interval 3
  note: Interval 2
  note: Interval 1
  note: zero
      | space vector
      | (Q1 Q3 Q5 =0)
  note: 1st basic
      | space vector
  note: 2nd basic
      | space vector
  note: zero
      | space vector
      | (Q1 Q3 Q5 =1)
  note: zero
      | space vector
      | (Q1 Q3 Q5 =0)
  note: 2nd basic
      | space vector
  note: 1st basic
      | space vector
  note: Pattern #1 implements the following symmetrical switching pattern:
      | total duration = 1 PWM period (Tpwm = 1/Fc)
  note: |
      | |
      | |
      | |
      | |
      | |
      | |
      | |
      | |
      | |
  note: |
      | |
      | |
      | |
      | |
      | |
      | |
      | |
      | |
      | |
  note: |
      | |
      | |
      | |
      | |
      | |
      | |
      | |
      | |
      | |
  note: |
      | |
      | |
      | |
      | |
      | |
      | |
      | |
      | |
      | |
  note: |
      | |
      | |
      | |
      | |
      | |
      | |
      | |
      | |
      | |
  note: |
      | |
      | |
      | |
      | |
      | |
      | |
      | |
      | |
      | |
  note: Ta/2
  note: To/4
  note: Tb/2
  note: To/2
  note: Tb/2
  note: Ta/2
  note: To/4
  note: Ta=m*cos(alpha+30)* (1/Fc)
  note: Tb=m*sin(alpha) * (1/Fc)
  note: To=(1/Fc-Ta-Tb)
  note: where:
      | Fc = Chopping frequency
      | m = modulation index
      | alpha = angle between reference vector U* and
      | 1st basic space vector
